simulink model "MotorPositionControl"  (R2020a)
settings: Solver=VariableStepAuto  StartTime=0.0  StopTime=0.05  RelTol=1e-3
PostLoadFcn:
  | J=3.2284e-6;
  | L=2.75e-6;
  | R=4;
  | Ke=0.0274;
  | Kt=0.0274;
  | b=3.5077e-6;
model workspace (MAT data in the model file):
  Kd = 0.146
  Ki = 244
  Kp = 21.61
  N = 1828
settings Model: DataDictionary=DataDicn.sldd  Creator=Hp  LastModifiedBy=Hp

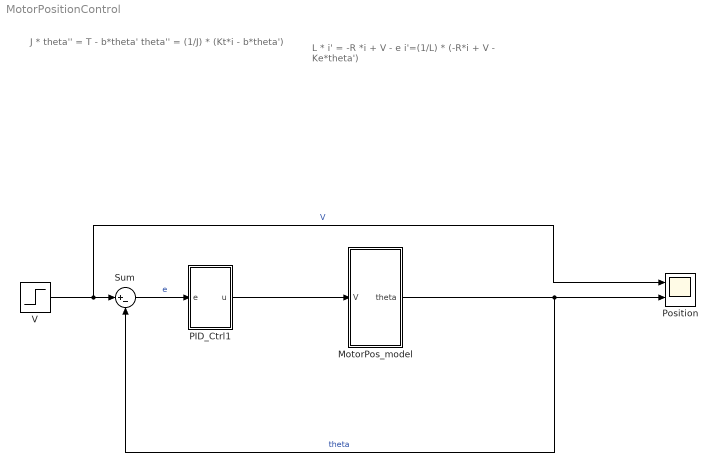
== system MotorPositionControl ==
  note: L * i' = -R *i + V - e
      | i'=(1/L) * (-R*i + V - Ke*theta')
  note: J * theta'' = T - b*theta'
      | theta'' = (1/J) * (Kt*i - b*theta')
  MotorPos_model : Subsystem
  PID_Ctrl1 : Subsystem
  Position : Scope  NumInputPorts=2
  Sum : Sum  Inputs=|+-
  V : Step  Time=0  SampleTime=0
  wires:
  MotorPos_model/1(theta) -> Sum/2, Position/2  "theta"
  V/1 -> Position/1, Sum/1  "V"
  Sum/1 -> PID_Ctrl1/1(e)  "e"
  PID_Ctrl1/1(u) -> MotorPos_model/1(V)

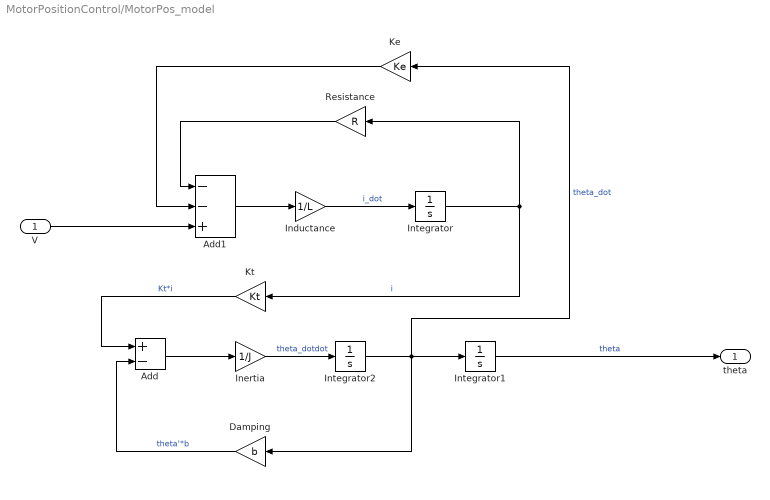
== system MotorPositionControl/MotorPos_model ==
  V : Inport
  Add : Sum  Inputs=+-
  Add1 : Sum  Inputs=--+
  Damping : Gain  Gain=b
  Inductance : Gain  Gain=1/L
  Inertia : Gain  Gain=1/J
  Integrator : Integrator
  Integrator1 : Integrator
  Integrator2 : Integrator
  Ke : Gain  Gain=Ke
  Kt : Gain  Gain=Kt
  Resistance : Gain  Gain=R
  theta : Outport
  wires:
  Kt/1 -> Add/1  "Kt*i"
  Inductance/1 -> Integrator/1  "i_dot"
  Add1/1 -> Inductance/1
  Damping/1 -> Add/2  "theta'*b"
  Integrator2/1 -> Damping/1, Integrator1/1, Ke/1  "theta_dot"
  Integrator/1 -> Resistance/1, Kt/1  "i"
  Inertia/1 -> Integrator2/1  "theta_dotdot"
  Integrator1/1 -> theta/1  "theta"
  V/1 -> Add1/3
  Add/1 -> Inertia/1
  Resistance/1 -> Add1/1
  Ke/1 -> Add1/2

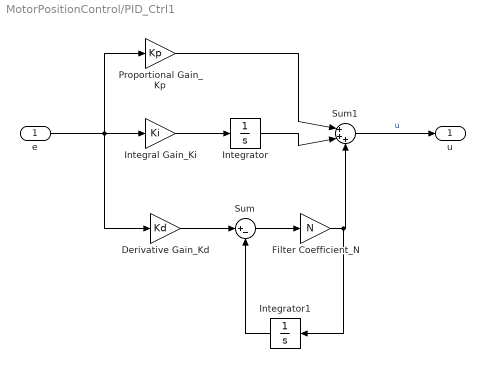
== system MotorPositionControl/PID_Ctrl1 ==
  e : Inport
  Derivative Gain_Kd : Gain  Gain=Kd
  Filter Coefficient_N : Gain  Gain=N
  Integral Gain_Ki : Gain  Gain=Ki
  Integrator : Integrator
  Integrator1 : Integrator
  Proportional Gain_Kp : Gain  Gain=Kp
  Sum : Sum  Inputs=|+-
  Sum1 : Sum  Inputs=|+++
  u : Outport
  wires:
  Integrator/1 -> Sum1/2
  Integral Gain_Ki/1 -> Integrator/1
  e/1 -> Integral Gain_Ki/1, Proportional Gain_Kp/1, Derivative Gain_Kd/1
  Proportional Gain_Kp/1 -> Sum1/1
  Sum1/1 -> u/1  "u"
  Derivative Gain_Kd/1 -> Sum/1
  Sum/1 -> Filter Coefficient_N/1
  Filter Coefficient_N/1 -> Integrator1/1, Sum1/3
  Integrator1/1 -> Sum/2
